simulink model "HeliControl_with_UDE_R2018a"  (Simulink 9.1)
settings: Solver=ode3  StartTime=0.0  StopTime=50  FixedStep=0.005  RelTol=1e-3
StopFcn:
  | %save('data.mat','ans_eps','ans_eps_d','ans_psi','ans_psi_d','ans_theta','ans_theta_d','u_ele','u_psi','u_theta','dhat_ele','dhat_psi','dhat_theta')
values from neighbouring files (symbols this model uses):
  a1 = 0.2634    [init_simulation.m]
  a2 = 1.6279    [init_simulation.m]
  a3 = 25.6488    [init_simulation.m]
  b1 = 0.531    [init_simulation.m]
  b2 = 5.3292    [init_simulation.m]
  b3 = 0.531    [init_simulation.m]
  b4 = 0.1157    [init_simulation.m]
  ce = 0.3010    (= 0.301)    [init_simulation.m]
  cp = 0.6804    [init_simulation.m]
  ct = 0.3410    (= 0.341)    [init_simulation.m]
  k_double_epsilon = [ ki_epsilon  kp_epsilon   kd_epsilon ]    [init_simulation.m]
  k_double_psi = [ki_psi   kp_psi    kd_psi]    [init_simulation.m]
  k_double_theta = [ki_theta   kp_theta   kd_theta]    [init_simulation.m]
  n = 0.9    [init_simulation.m]
  w = 125.66    [init_simulation.m]
undefined symbols (not defined in the file or in its folder): epsilon_T, psi_T, theta_T
libraries: powerlib_extras x1
settings Model: Creator=5420  LastModifiedBy=LaVie  ExtModeTrigDuration=200000
settings DataIOCC: LimitDataPoints=on  SignalLoggingSaveFormat=ModelDataLogs  SignalLoggingName=sigsOut
settings OptimizationCC: ExpressionDepthLimit=2147483647  InitFltsAndDblsToZero=on  LifeSpan=auto
settings DebuggingCC: SaveWithParameterizedLinksMsg=none  SignalResolutionControl=TryResolveAllWithWarning  MultiTaskDSMMsg=warning  MultiTaskCondExecSysMsg=none  StateNameClashWarn=warning
settings HardwareCC: ProdBitPerLong=64  ProdBitPerPointer=64  ProdBitPerSizeT=64  ProdBitPerPtrDiffT=64  ProdLargestAtomicFloat=Float  ProdIntDivRoundTo=Zero  ProdEndianess=LittleEndian  ProdWordSize=64  ProdHWDeviceType=Intel->x86-64 (Linux 64)
settings RTWCC: Description=Simulink Desktop Real-Time  SystemTargetFile=sldrt.tlc  TemplateMakefile=sldrt.tmf  RTWCompilerOptimization=on
settings CodeAppCC: MaxIdLength=95
settings SimulinkDesktopRealTimeCC: TargetLibSuffix=_sldrt.a  TargetPreCompLibLocation=E:\matlab2022a\toolbox\sldrt\lib\win64  TargetLangStandard=C89/C90 (ANSI)  ModelReferenceCompliant=off  CompOptLevelCompliant=off  SupportVariableSizeSignals=off

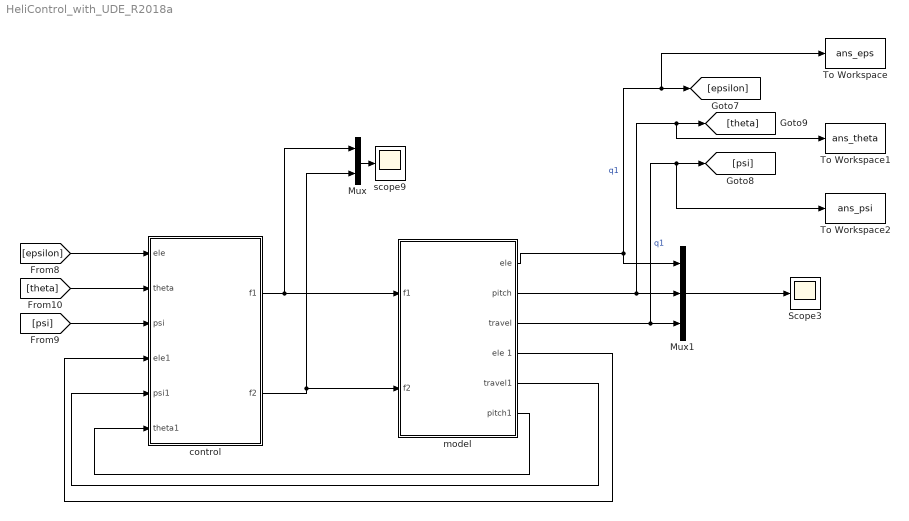
== system HeliControl_with_UDE_R2018a ==
  Mux : Mux  Inputs=2
  Mux1 : Mux  Inputs=3
  Scope3 : Scope
  To Workspace : ToWorkspace  VariableName=ans_eps  SaveFormat=Structure With Time  SampleTime=-1
      settings: Save2DSignal=2-D array (concatenate along first dimension)
  To Workspace1 : ToWorkspace  VariableName=ans_theta  SampleTime=-1
      settings: Save2DSignal=2-D array (concatenate along first dimension)
  To Workspace2 : ToWorkspace  VariableName=ans_psi  SampleTime=-1
      settings: Save2DSignal=2-D array (concatenate along first dimension)
  control : Subsystem
  model : Subsystem
  scope9 : Scope
  wires:
  Mux1/1 -> Scope3/1
  control/2(f2) -> Mux/2, model/2(f2)
  control/1(f1) -> Mux/1, model/1(f1)
  [epsilon] -> control/1(ele)
  [theta] -> control/2(theta)
  [psi] -> control/3(psi)
  Mux/1 -> scope9/1
  model/1("ele ") -> To Workspace/1, [epsilon], Mux1/1  "q1"
  model/2(pitch) -> To Workspace1/1, [theta], Mux1/2
  model/3(travel) -> To Workspace2/1, [psi], Mux1/3  "q1"
  model/4(ele 1) -> control/4(ele1)
  model/5(travel1) -> control/5(psi1)
  model/6(pitch1) -> control/6(theta1)

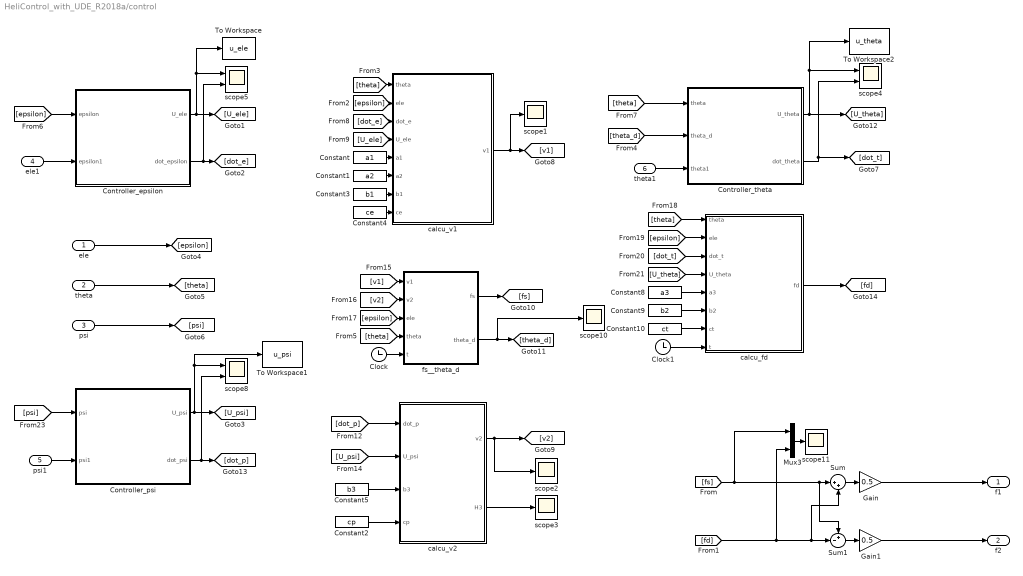
== system HeliControl_with_UDE_R2018a/control ==
  ele : Inport
  theta : Inport  Port=2
  psi : Inport  Port=3
  ele1 : Inport  Port=4
  psi1 : Inport  Port=5
  theta1 : Inport  Port=6
  Clock : Clock
      settings: Decimation=30
  Clock1 : Clock
      settings: Decimation=30
  Constant : Constant  Value=a1
  Constant1 : Constant  Value=a2
  Constant10 : Constant  Value=ct
  Constant2 : Constant  Value=cp
  Constant3 : Constant  Value=b1
  Constant4 : Constant  Value=ce
  Constant5 : Constant  Value=b3
  Constant8 : Constant  Value=a3
  Constant9 : Constant  Value=b2
  Controller_epsilon : Subsystem
  Controller_psi : Subsystem
  Controller_theta : Subsystem
  Gain : Gain  Gain=0.5
  Gain1 : Gain  Gain=0.5
  Mux3 : Mux  Inputs=2
  Sum : Sum  Inputs=|++
  Sum1 : Sum  Inputs=+-|
  To Workspace : ToWorkspace  VariableName=u_ele  SampleTime=-1
      settings: Save2DSignal=2-D array (concatenate along first dimension)
  To Workspace1 : ToWorkspace  VariableName=u_psi  SampleTime=-1
      settings: Save2DSignal=2-D array (concatenate along first dimension)
  To Workspace2 : ToWorkspace  VariableName=u_theta  SampleTime=-1
      settings: Save2DSignal=2-D array (concatenate along first dimension)
  calcu_fd : MATLAB Function  TreatAsAtomicUnit=on
  calcu_v1 : MATLAB Function  TreatAsAtomicUnit=on
  calcu_v2 : MATLAB Function  TreatAsAtomicUnit=on
  fs__theta_d : MATLAB Function  TreatAsAtomicUnit=on
  scope{1..3,10..11} (5 alike) : Scope
  scope4 : Scope  NumInputPorts=2
  scope5 : Scope  NumInputPorts=2
  scope8 : Scope  NumInputPorts=2
  f1 : Outport  VectorParamsAs1DForOutWhenUnconnected=off
  f2 : Outport  Port=2  VectorParamsAs1DForOutWhenUnconnected=off
  wires:
  [theta] -> calcu_v1/1(theta)
  [epsilon] -> calcu_v1/2(ele)
  calcu_v2/1(v2) -> [v2], scope2/1
  [U_ele] -> calcu_v1/4(U_ele)
  [dot_e] -> calcu_v1/3(dot_e)
  calcu_v1/1(v1) -> scope1/1, [v1]
  [v1] -> fs__theta_d/1(v1)
  [v2] -> fs__theta_d/2(v2)
  [epsilon] -> fs__theta_d/3(ele)
  fs__theta_d/1(fs) -> [fs]
  fs__theta_d/2(theta_d) -> scope10/1, [theta_d]
  [theta] -> calcu_fd/1(theta)
  [epsilon] -> calcu_fd/2(ele)
  [dot_t] -> calcu_fd/3(dot_t)
  [U_theta] -> calcu_fd/4(U_theta)
  calcu_fd/1(fd) -> [fd]
  [fd] -> Sum/2, Sum1/2, Mux3/2
  Sum/1 -> Gain/1
  Sum1/1 -> Gain1/1
  ele/1 -> [epsilon]
  theta/1 -> [theta]
  psi/1 -> [psi]
  Mux3/1 -> scope11/1
  Constant/1 -> calcu_v1/5(a1)
  Constant1/1 -> calcu_v1/6(a2)
  Constant3/1 -> calcu_v1/7(b1)
  Constant4/1 -> calcu_v1/8(ce)
  Constant8/1 -> calcu_fd/5(a3)
  Constant9/1 -> calcu_fd/6(b2)
  Constant10/1 -> calcu_fd/7(ct)
  [theta] -> fs__theta_d/4(theta)
  Clock/1 -> fs__theta_d/5(t)
  Clock1/1 -> calcu_fd/8(t)
  calcu_v2/2(H3) -> scope3/1
  [epsilon] -> Controller_epsilon/1(epsilon)
  Controller_epsilon/2(dot_epsilon) -> scope5/2, [dot_e]
  [psi] -> Controller_psi/1(psi)
  Controller_psi/1(U_psi) -> scope8/1, To Workspace1/1, [U_psi]
  Controller_psi/2(dot_psi) -> scope8/2, [dot_p]
  [theta] -> Controller_theta/1(theta)
  Controller_theta/1(U_theta) -> To Workspace2/1, scope4/1, [U_theta]
  Controller_theta/2(dot_theta) -> scope4/2, [dot_t]
  [theta_d] -> Controller_theta/2(theta_d)
  Controller_epsilon/1(U_ele) -> To Workspace/1, scope5/1, [U_ele]
  ele1/1 -> Controller_epsilon/2(epsilon1)
  psi1/1 -> Controller_psi/2(psi1)
  theta1/1 -> Controller_theta/3(theta1)
  Gain/1 -> f1/1
  Gain1/1 -> f2/1
  [fs] -> Sum1/1, Sum/1, Mux3/1
  [dot_p] -> calcu_v2/1(dot_p)
  [U_psi] -> calcu_v2/2(U_psi)
  Constant5/1 -> calcu_v2/3(b3)
  Constant2/1 -> calcu_v2/4(cp)

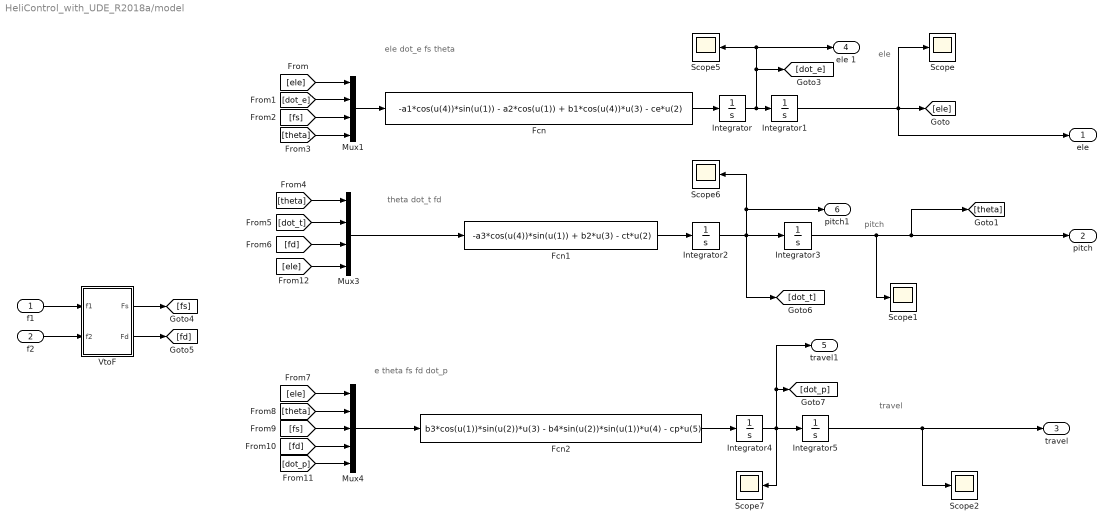
== system HeliControl_with_UDE_R2018a/model ==
  note: e
      | theta
      | fs
      | fd
      | dot_p
  note: ele
      | dot_e
      | fs
      | theta
  note: travel
  note: pitch
  note: ele
  note: theta
      | dot_t
      | fd
  f1 : Inport
  f2 : Inport  Port=2
  Fcn : Fcn  Expr=-a1*cos(u(4))*sin(u(1)) - a2*cos(u(1)) + b1*cos(u(4))*u(3) - ce*u(2)
  Fcn1 : Fcn  Expr=-a3*cos(u(4))*sin(u(1)) + b2*u(3) - ct*u(2)
  Fcn2 : Fcn  Expr=b3*cos(u(1))*sin(u(2))*u(3) - b4*sin(u(2))*sin(u(1))*u(4) - cp*u(5)
  Integrator{,2..5} (5 alike) : Integrator
  Integrator1 : Integrator  InitialCondition=-0.713
  Mux1 : Mux
  Mux3 : Mux
  Mux4 : Mux  Inputs=5
  Scope{,1..2,5..7} (6 alike) : Scope
  VtoF : Subsystem
  "ele " : Outport  VectorParamsAs1DForOutWhenUnconnected=off
  pitch : Outport  Port=2  VectorParamsAs1DForOutWhenUnconnected=off
  travel : Outport  Port=3  VectorParamsAs1DForOutWhenUnconnected=off
  ele 1 : Outport  Port=4  VectorParamsAs1DForOutWhenUnconnected=off
  travel1 : Outport  Port=5  VectorParamsAs1DForOutWhenUnconnected=off
  pitch1 : Outport  Port=6  VectorParamsAs1DForOutWhenUnconnected=off
  wires:
  Integrator1/1 -> "ele "/1, Scope/1, [ele]
  Fcn/1 -> Integrator/1
  Integrator3/1 -> pitch/1, [theta], Scope1/1
  Integrator/1 -> ele 1/1, Scope5/1, [dot_e], Integrator1/1
  Fcn1/1 -> Integrator2/1
  Fcn2/1 -> Integrator4/1
  Integrator4/1 -> Scope7/1, travel1/1, [dot_p], Integrator5/1
  Integrator5/1 -> travel/1, Scope2/1
  Mux1/1 -> Fcn/1
  Mux4/1 -> Fcn2/1
  [ele] -> Mux1/1
  [dot_e] -> Mux1/2
  VtoF/1(Fs) -> [fs]
  VtoF/2(Fd) -> [fd]
  [fs] -> Mux1/3
  [theta] -> Mux1/4
  [ele] -> Mux4/1
  [theta] -> Mux4/2
  [fs] -> Mux4/3
  [fd] -> Mux4/4
  [dot_p] -> Mux4/5
  Integrator2/1 -> Scope6/1, pitch1/1, [dot_t], Integrator3/1
  f1/1 -> VtoF/1(f1)
  f2/1 -> VtoF/2(f2)
  Mux3/1 -> Fcn1/1
  [theta] -> Mux3/1
  [dot_t] -> Mux3/2
  [fd] -> Mux3/3
  [ele] -> Mux3/4

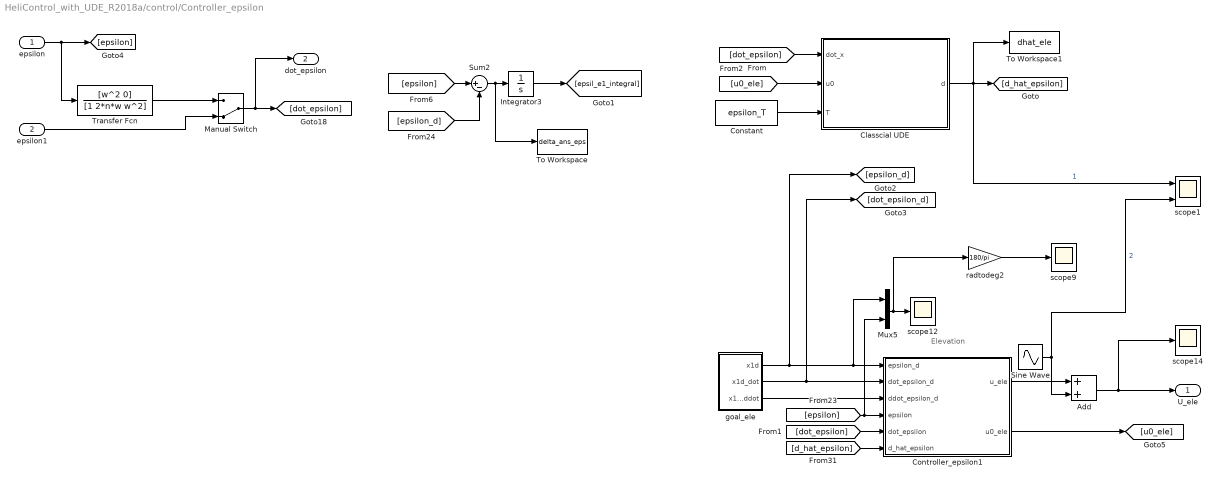
== system HeliControl_with_UDE_R2018a/control/Controller_epsilon ==
  note: Elevation
  epsilon : Inport
  epsilon1 : Inport  Port=2
  Add : Sum
  Classcial UDE : Subsystem
  Constant : Constant  Value=epsilon_T  VectorParams1D=off  SampleTime=-1
  Controller_epsilon1 : Subsystem
  Integrator3 : Integrator
  Manual Switch : ManualSwitch  CurrentSetting=0
  Mux5 : Mux  Inputs=2
  Sine Wave : Sin  Amplitude=0.05  Bias=0.1  Frequency=0.5  SampleTime=0
  Sum2 : Sum  Inputs=|+-
  To Workspace : ToWorkspace  VariableName=delta_ans_eps  SaveFormat=Timeseries  SampleTime=-1
  To Workspace1 : ToWorkspace  VariableName=dhat_ele  SampleTime=-1
      settings: Save2DSignal=2-D array (concatenate along first dimension)
  Transfer Fcn : TransferFcn  Numerator=[w^2 0]  Denominator=[1 2*n*w w^2]
  goal_ele : Subsystem
  radtodeg2 : Gain  Gain=180/pi
  scope1 : Scope  NumInputPorts=2
  scope12 : Scope
  scope14 : Scope
  scope9 : Scope
  U_ele : Outport  VectorParamsAs1DForOutWhenUnconnected=off
  dot_epsilon : Outport  Port=2  VectorParamsAs1DForOutWhenUnconnected=off
  wires:
  [epsilon] -> Controller_epsilon1/4(epsilon), Mux5/2
  Mux5/1 -> radtodeg2/1, scope12/1
  Add/1 -> scope14/1, U_ele/1
  radtodeg2/1 -> scope9/1
  goal_ele/1(x1d) -> Mux5/1, Controller_epsilon1/1(epsilon_d), [epsilon_d]
  goal_ele/2(x1d_dot) -> [dot_epsilon_d], Controller_epsilon1/2(dot_epsilon_d)
  goal_ele/3(x1d_ddot) -> Controller_epsilon1/3(ddot_epsilon_d)
  Sum2/1 -> To Workspace/1, Integrator3/1
  Integrator3/1 -> [epsil_e1_integral]
  [epsilon_d] -> Sum2/2
  [epsilon] -> Sum2/1
  [d_hat_epsilon] -> Controller_epsilon1/6(d_hat_epsilon)
  epsilon/1 -> Transfer Fcn/1, [epsilon]
  [dot_epsilon] -> Controller_epsilon1/5(dot_epsilon)
  Transfer Fcn/1 -> Manual Switch/1
  Manual Switch/1 -> dot_epsilon/1, [dot_epsilon]
  epsilon1/1 -> Manual Switch/2
  Controller_epsilon1/2(u0_ele) -> [u0_ele]
  Classcial UDE/1(d) -> scope1/1, To Workspace1/1, [d_hat_epsilon]  "1"
  [dot_epsilon] -> Classcial UDE/1(dot_x)
  [u0_ele] -> Classcial UDE/2(u0)
  Constant/1 -> Classcial UDE/3(T)
  Controller_epsilon1/1(u_ele) -> Add/1
  Sine Wave/1 -> Add/2, scope1/2  "2"

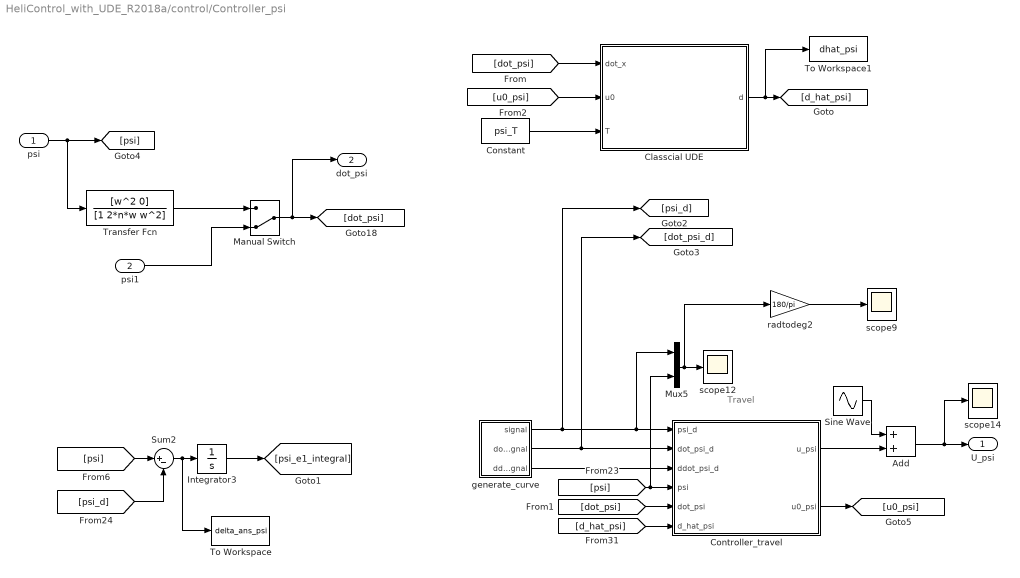
== system HeliControl_with_UDE_R2018a/control/Controller_psi ==
  note: Travel
  psi : Inport
  psi1 : Inport  Port=2
  Add : Sum
  Classcial UDE : Subsystem
  Constant : Constant  Value=psi_T  VectorParams1D=off  SampleTime=-1
  Controller_travel : Subsystem
  Integrator3 : Integrator
  Manual Switch : ManualSwitch  CurrentSetting=0
  Mux5 : Mux  Inputs=2
  Sine Wave : Sin  Amplitude=0.05  Bias=0.1  Frequency=2  SampleTime=0
  Sum2 : Sum  Inputs=|+-
  To Workspace : ToWorkspace  VariableName=delta_ans_psi  SaveFormat=Timeseries  SampleTime=-1
  To Workspace1 : ToWorkspace  VariableName=dhat_psi  SampleTime=-1
      settings: Save2DSignal=2-D array (concatenate along first dimension)
  Transfer Fcn : TransferFcn  Numerator=[w^2 0]  Denominator=[1 2*n*w w^2]
  generate_curve : Subsystem
  radtodeg2 : Gain  Gain=180/pi
  scope12 : Scope
  scope14 : Scope
  scope9 : Scope
  U_psi : Outport  VectorParamsAs1DForOutWhenUnconnected=off
  dot_psi : Outport  Port=2  VectorParamsAs1DForOutWhenUnconnected=off
  wires:
  [psi] -> Controller_travel/4(psi), Mux5/2
  Mux5/1 -> radtodeg2/1, scope12/1
  Add/1 -> U_psi/1, scope14/1
  radtodeg2/1 -> scope9/1
  generate_curve/1(signal) -> Mux5/1, Controller_travel/1(psi_d), [psi_d]
  generate_curve/2(dot_signal) -> [dot_psi_d], Controller_travel/2(dot_psi_d)
  generate_curve/3(ddot_signal) -> Controller_travel/3(ddot_psi_d)
  Sum2/1 -> To Workspace/1, Integrator3/1
  Integrator3/1 -> [psi_e1_integral]
  [psi_d] -> Sum2/2
  [psi] -> Sum2/1
  [d_hat_psi] -> Controller_travel/6(d_hat_psi)
  psi/1 -> Transfer Fcn/1, [psi]
  [dot_psi] -> Controller_travel/5(dot_psi)
  Transfer Fcn/1 -> Manual Switch/1
  Manual Switch/1 -> dot_psi/1, [dot_psi]
  psi1/1 -> Manual Switch/2
  [dot_psi] -> Classcial UDE/1(dot_x)
  Classcial UDE/1(d) -> To Workspace1/1, [d_hat_psi]
  [u0_psi] -> Classcial UDE/2(u0)
  Constant/1 -> Classcial UDE/3(T)
  Controller_travel/2(u0_psi) -> [u0_psi]
  Sine Wave/1 -> Add/1
  Controller_travel/1(u_psi) -> Add/2

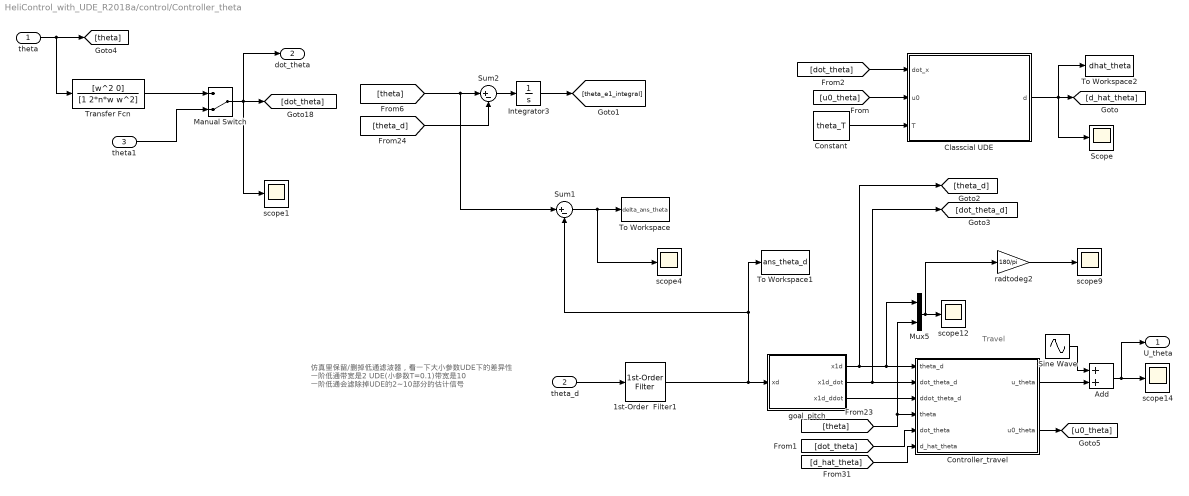
== system HeliControl_with_UDE_R2018a/control/Controller_theta ==
  note: 仿真里保留/删掉低通滤波器，看一下大小参数UDE下的差异性
      | 一阶低通带宽是2
      | UDE(小参数T=0.1)带宽是10
      | 一阶低通会滤除掉UDE的2~10部分的估计信号
  note: Travel
  theta : Inport
  theta_d : Inport  Port=2
  theta1 : Inport  Port=3
  1st-Order  Filter1 : powerlib_extras/Control  Blocks/1st-Order  Filter  FilterType=Lowpass  Tc=0.5  Initialize=off  Vac_Init=[0.8 -25 60]  Vdc_Init=-0.4  PlotResponse=off  param1=[1 500 1]
      settings: SourceProductBaseCode=PS
  Add : Sum
  Classcial UDE : Subsystem
  Constant : Constant  Value=theta_T  VectorParams1D=off  SampleTime=-1
  Controller_travel : Subsystem
  Integrator3 : Integrator
  Manual Switch : ManualSwitch  CurrentSetting=0
  Mux5 : Mux  Inputs=2
  Scope : Scope
  Sine Wave : Sin  Amplitude=0.05  Bias=0.1  Frequency=5  SampleTime=0
  Sum1 : Sum  Inputs=|+-
  Sum2 : Sum  Inputs=|+-
  To Workspace : ToWorkspace  VariableName=delta_ans_theta  SaveFormat=Timeseries  SampleTime=-1
  To Workspace1 : ToWorkspace  VariableName=ans_theta_d  SampleTime=-1
      settings: Save2DSignal=2-D array (concatenate along first dimension)
  To Workspace2 : ToWorkspace  VariableName=dhat_theta  SampleTime=-1
      settings: Save2DSignal=2-D array (concatenate along first dimension)
  Transfer Fcn : TransferFcn  Numerator=[w^2 0]  Denominator=[1 2*n*w w^2]
  goal_pitch : Subsystem
  radtodeg2 : Gain  Gain=180/pi
  scope{1,4,9,12,14} (5 alike) : Scope
  U_theta : Outport  VectorParamsAs1DForOutWhenUnconnected=off
  dot_theta : Outport  Port=2  VectorParamsAs1DForOutWhenUnconnected=off
  wires:
  [theta] -> Controller_travel/4(theta), Mux5/2
  Mux5/1 -> radtodeg2/1, scope12/1
  Add/1 -> scope14/1, U_theta/1
  radtodeg2/1 -> scope9/1
  goal_pitch/1(x1d) -> Mux5/1, Controller_travel/1(theta_d), [theta_d]
  goal_pitch/2(x1d_dot) -> [dot_theta_d], Controller_travel/2(dot_theta_d)
  goal_pitch/3(x1d_ddot) -> Controller_travel/3(ddot_theta_d)
  Sum2/1 -> Integrator3/1
  Integrator3/1 -> [theta_e1_integral]
  [theta_d] -> Sum2/2
  [d_hat_theta] -> Controller_travel/6(d_hat_theta)
  theta/1 -> Transfer Fcn/1, [theta]
  [dot_theta] -> Controller_travel/5(dot_theta)
  Transfer Fcn/1 -> Manual Switch/1
  Manual Switch/1 -> scope1/1, dot_theta/1, [dot_theta]
  theta1/1 -> Manual Switch/2
  [theta] -> Sum1/1, Sum2/1
  Sum1/1 -> scope4/1, To Workspace/1
  1st-Order  Filter1/1 -> goal_pitch/1(xd), To Workspace1/1, Sum1/2
  Controller_travel/2(u0_theta) -> [u0_theta]
  [u0_theta] -> Classcial UDE/2(u0)
  Classcial UDE/1(d) -> Scope/1, To Workspace2/1, [d_hat_theta]
  [dot_theta] -> Classcial UDE/1(dot_x)
  Constant/1 -> Classcial UDE/3(T)
  Sine Wave/1 -> Add/1
  Controller_travel/1(u_theta) -> Add/2
  theta_d/1 -> 1st-Order  Filter1/1

== system HeliControl_with_UDE_R2018a/model/VtoF ==
  f1 : Inport
  f2 : Inport  Port=2
  Add : Sum
  Add1 : Sum  Inputs=+-
  Fs : Outport  VectorParamsAs1DForOutWhenUnconnected=off
  Fd : Outport  Port=2  VectorParamsAs1DForOutWhenUnconnected=off
  wires:
  Add1/1 -> Fd/1
  f2/1 -> Add1/2, Add/2
  f1/1 -> Add1/1, Add/1
  Add/1 -> Fs/1

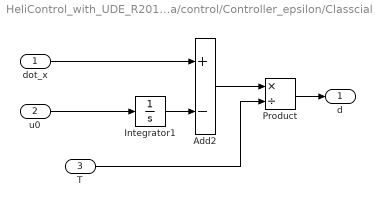
== system HeliControl_with_UDE_R2018a/control/Controller_epsilon/Classcial UDE ==
  dot_x : Inport
  u0 : Inport  Port=2
  T : Inport  Port=3
  Add2 : Sum  Inputs=+-
  Integrator1 : Integrator
  Product : Product  Inputs=*/
  d : Outport  VectorParamsAs1DForOutWhenUnconnected=off
  wires:
  dot_x/1 -> Add2/1
  Integrator1/1 -> Add2/2
  u0/1 -> Integrator1/1
  Add2/1 -> Product/1
  Product/1 -> d/1
  T/1 -> Product/2

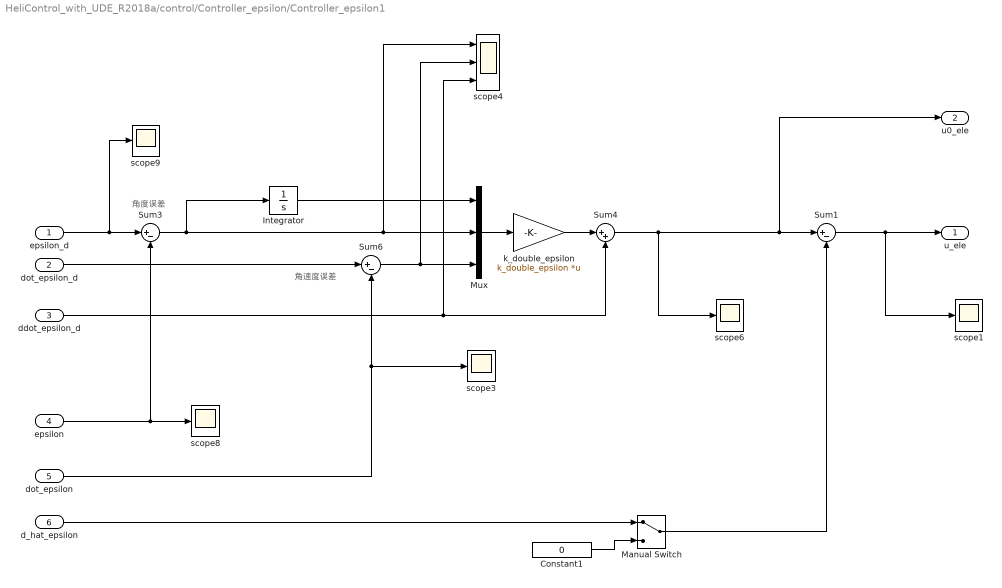
== system HeliControl_with_UDE_R2018a/control/Controller_epsilon/Controller_epsilon1 ==
  note: 角速度误差
  note: 角度误差
  epsilon_d : Inport
  dot_epsilon_d : Inport  Port=2
  ddot_epsilon_d : Inport  Port=3
  epsilon : Inport  Port=4
  dot_epsilon : Inport  Port=5
  d_hat_epsilon : Inport  Port=6
  Constant1 : Constant  Value=0
  Integrator : Integrator
  Manual Switch : ManualSwitch
  Mux : Mux  Inputs=3
  Sum1 : Sum  Inputs=|+-
  Sum3 : Sum  Inputs=|+-
  Sum4 : Sum  Inputs=|++
  Sum6 : Sum  Inputs=|+-
  k_double_epsilon : Gain  Gain=k_double_epsilon  Multiplication=Matrix(K*u)
  scope{1,3,6,8..9} (5 alike) : Scope
  scope4 : Scope  NumInputPorts=3
  u_ele : Outport  VectorParamsAs1DForOutWhenUnconnected=off
  u0_ele : Outport  Port=2  VectorParamsAs1DForOutWhenUnconnected=off
  wires:
  epsilon/1 -> Sum3/2, scope8/1
  epsilon_d/1 -> scope9/1, Sum3/1
  Sum4/1 -> u0_ele/1, Sum1/1, scope6/1
  Sum3/1 -> scope4/1, Mux/2, Integrator/1
  Sum6/1 -> scope4/2, Mux/3
  Mux/1 -> k_double_epsilon/1
  dot_epsilon_d/1 -> Sum6/1
  k_double_epsilon/1 -> Sum4/1
  ddot_epsilon_d/1 -> scope4/3, Sum4/2
  dot_epsilon/1 -> Sum6/2, scope3/1
  Integrator/1 -> Mux/1
  Sum1/1 -> scope1/1, u_ele/1
  Manual Switch/1 -> Sum1/2
  d_hat_epsilon/1 -> Manual Switch/1
  Constant1/1 -> Manual Switch/2

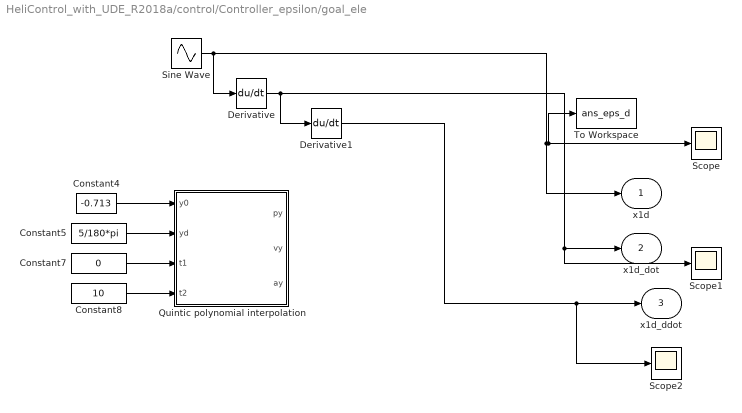
== system HeliControl_with_UDE_R2018a/control/Controller_epsilon/goal_ele ==
  Constant4 : Constant  Value=-0.713  VectorParams1D=off  SampleTime=-1
  Constant5 : Constant  Value=5/180*pi  VectorParams1D=off  SampleTime=-1
  Constant7 : Constant  Value=0  VectorParams1D=off  SampleTime=-1
  Constant8 : Constant  Value=10  VectorParams1D=off  SampleTime=-1
  Derivative : Derivative
  Derivative1 : Derivative
  Quintic polynomial interpolation : Subsystem
  Scope : Scope
  Scope1 : Scope
  Scope2 : Scope
  Sine Wave : Sin  Amplitude=-2*pi/180  Bias=2*pi/180  Frequency=0.4*pi  Phase=pi/2  SampleTime=0
  To Workspace : ToWorkspace  VariableName=ans_eps_d  SampleTime=-1
      settings: Save2DSignal=2-D array (concatenate along first dimension)
  x1d : Outport  VectorParamsAs1DForOutWhenUnconnected=off
  x1d_dot : Outport  Port=2  VectorParamsAs1DForOutWhenUnconnected=off
  x1d_ddot : Outport  Port=3  VectorParamsAs1DForOutWhenUnconnected=off
  wires:
  Derivative1/1 -> Scope2/1, x1d_ddot/1
  Derivative/1 -> Derivative1/1, Scope1/1, x1d_dot/1
  Sine Wave/1 -> Derivative/1, x1d/1, To Workspace/1, Scope/1
  Constant4/1 -> Quintic polynomial interpolation/1(y0)
  Constant5/1 -> Quintic polynomial interpolation/2(yd)
  Constant7/1 -> Quintic polynomial interpolation/3(t1)
  Constant8/1 -> Quintic polynomial interpolation/4(t2)

== system HeliControl_with_UDE_R2018a/control/Controller_psi/Classcial UDE ==
  dot_x : Inport
  u0 : Inport  Port=2
  T : Inport  Port=3
  Add2 : Sum  Inputs=+-
  Integrator1 : Integrator
  Product : Product  Inputs=*/
  d : Outport  VectorParamsAs1DForOutWhenUnconnected=off
  wires:
  dot_x/1 -> Add2/1
  Integrator1/1 -> Add2/2
  u0/1 -> Integrator1/1
  Add2/1 -> Product/1
  Product/1 -> d/1
  T/1 -> Product/2

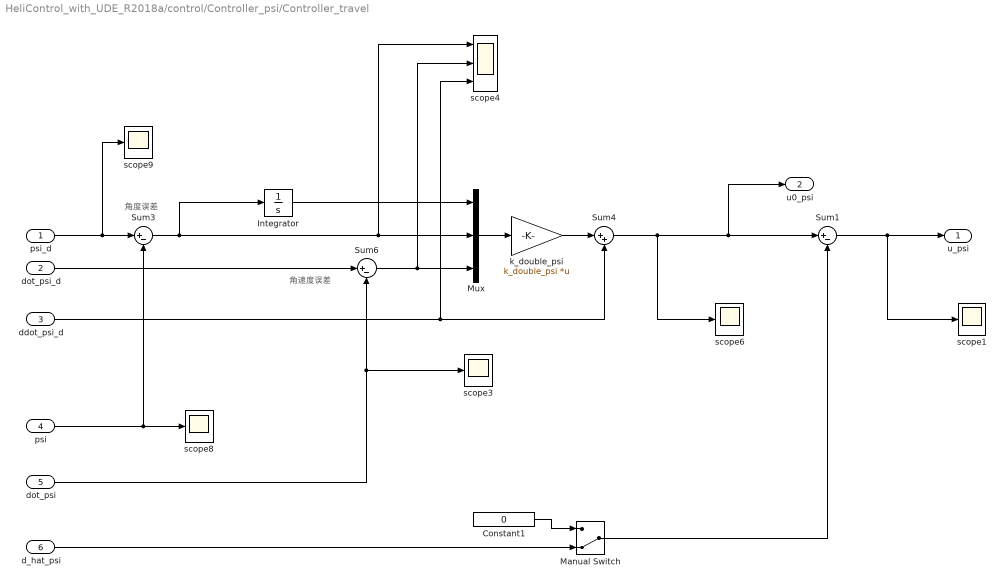
== system HeliControl_with_UDE_R2018a/control/Controller_psi/Controller_travel ==
  note: 角速度误差
  note: 角度误差
  psi_d : Inport
  dot_psi_d : Inport  Port=2
  ddot_psi_d : Inport  Port=3
  psi : Inport  Port=4
  dot_psi : Inport  Port=5
  d_hat_psi : Inport  Port=6
  Constant1 : Constant  Value=0
  Integrator : Integrator
  Manual Switch : ManualSwitch  CurrentSetting=0
  Mux : Mux  Inputs=3
  Sum1 : Sum  Inputs=|+-
  Sum3 : Sum  Inputs=|+-
  Sum4 : Sum  Inputs=|++
  Sum6 : Sum  Inputs=|+-
  k_double_psi : Gain  Gain=k_double_psi  Multiplication=Matrix(K*u)
  scope{1,3,6,8..9} (5 alike) : Scope
  scope4 : Scope  NumInputPorts=3
  u_psi : Outport  VectorParamsAs1DForOutWhenUnconnected=off
  u0_psi : Outport  Port=2  VectorParamsAs1DForOutWhenUnconnected=off
  wires:
  psi/1 -> Sum3/2, scope8/1
  psi_d/1 -> scope9/1, Sum3/1
  Sum4/1 -> u0_psi/1, Sum1/1, scope6/1
  Sum3/1 -> scope4/1, Mux/2, Integrator/1
  Sum6/1 -> scope4/2, Mux/3
  Mux/1 -> k_double_psi/1
  dot_psi_d/1 -> Sum6/1
  k_double_psi/1 -> Sum4/1
  ddot_psi_d/1 -> scope4/3, Sum4/2
  dot_psi/1 -> Sum6/2, scope3/1
  Integrator/1 -> Mux/1
  Sum1/1 -> scope1/1, u_psi/1
  Constant1/1 -> Manual Switch/1
  d_hat_psi/1 -> Manual Switch/2
  Manual Switch/1 -> Sum1/2

== system HeliControl_with_UDE_R2018a/control/Controller_psi/generate_curve ==
  Clock : Clock
  Constant1 : Constant  Value=0  VectorParams1D=off  SampleTime=-1
  MATLAB Function : MATLAB Function  TreatAsAtomicUnit=on
  To Workspace : ToWorkspace  VariableName=ans_psi_d  SampleTime=-1
      settings: Save2DSignal=2-D array (concatenate along first dimension)
  signal : Outport  VectorParamsAs1DForOutWhenUnconnected=off
  dot_signal : Outport  Port=2  VectorParamsAs1DForOutWhenUnconnected=off
  ddot_signal : Outport  Port=3  VectorParamsAs1DForOutWhenUnconnected=off
  wires:
  MATLAB Function/1(p) -> To Workspace/1, signal/1
  MATLAB Function/2(v) -> dot_signal/1
  Constant1/1 -> ddot_signal/1
  Clock/1 -> MATLAB Function/1(t)

== system HeliControl_with_UDE_R2018a/control/Controller_theta/Classcial UDE ==
  dot_x : Inport
  u0 : Inport  Port=2
  T : Inport  Port=3
  Add2 : Sum  Inputs=+-
  Integrator1 : Integrator
  Product : Product  Inputs=*/
  d : Outport  VectorParamsAs1DForOutWhenUnconnected=off
  wires:
  dot_x/1 -> Add2/1
  Integrator1/1 -> Add2/2
  u0/1 -> Integrator1/1
  Add2/1 -> Product/1
  Product/1 -> d/1
  T/1 -> Product/2

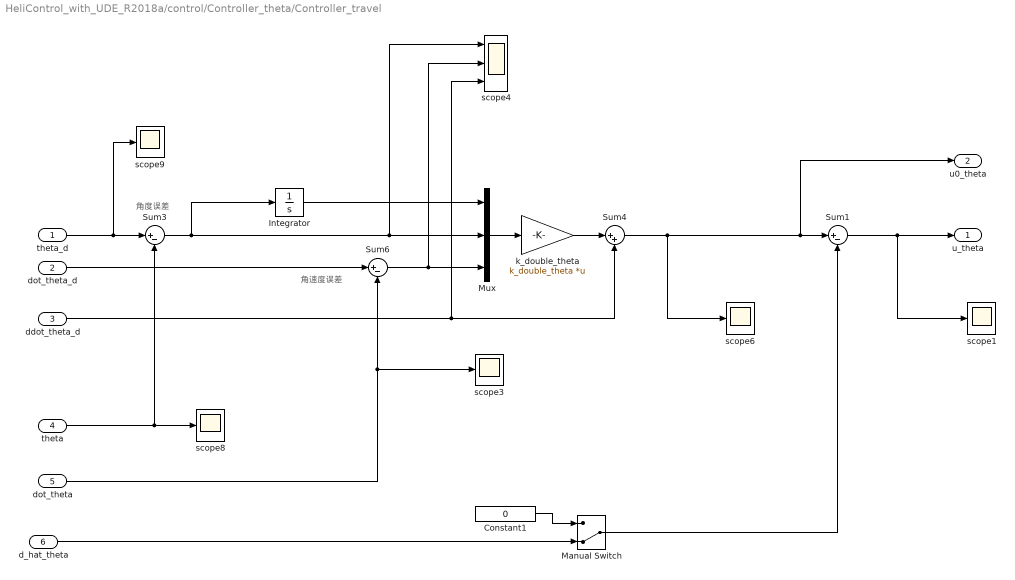
== system HeliControl_with_UDE_R2018a/control/Controller_theta/Controller_travel ==
  note: 角速度误差
  note: 角度误差
  theta_d : Inport
  dot_theta_d : Inport  Port=2
  ddot_theta_d : Inport  Port=3
  theta : Inport  Port=4
  dot_theta : Inport  Port=5
  d_hat_theta : Inport  Port=6
  Constant1 : Constant  Value=0
  Integrator : Integrator
  Manual Switch : ManualSwitch  CurrentSetting=0
  Mux : Mux  Inputs=3
  Sum1 : Sum  Inputs=|+-
  Sum3 : Sum  Inputs=|+-
  Sum4 : Sum  Inputs=|++
  Sum6 : Sum  Inputs=|+-
  k_double_theta : Gain  Gain=k_double_theta  Multiplication=Matrix(K*u)
  scope{1,3,6,8..9} (5 alike) : Scope
  scope4 : Scope  NumInputPorts=3
  u_theta : Outport  VectorParamsAs1DForOutWhenUnconnected=off
  u0_theta : Outport  Port=2
  wires:
  theta/1 -> Sum3/2, scope8/1
  theta_d/1 -> scope9/1, Sum3/1
  Sum4/1 -> u0_theta/1, Sum1/1, scope6/1
  Sum3/1 -> scope4/1, Mux/2, Integrator/1
  Sum6/1 -> scope4/2, Mux/3
  Mux/1 -> k_double_theta/1
  dot_theta_d/1 -> Sum6/1
  k_double_theta/1 -> Sum4/1
  ddot_theta_d/1 -> scope4/3, Sum4/2
  dot_theta/1 -> Sum6/2, scope3/1
  Integrator/1 -> Mux/1
  Sum1/1 -> scope1/1, u_theta/1
  Constant1/1 -> Manual Switch/1
  d_hat_theta/1 -> Manual Switch/2
  Manual Switch/1 -> Sum1/2

== system HeliControl_with_UDE_R2018a/control/Controller_theta/goal_pitch ==
  xd : Inport
  Transfer Fcn1 : TransferFcn  Numerator=[w^2 0]  Denominator=[1 2*n*w w^2]
  Transfer Fcn2 : TransferFcn  Numerator=[w^2 0]  Denominator=[1 2*n*w w^2]
  scope1 : Scope
  x1d : Outport  VectorParamsAs1DForOutWhenUnconnected=off
  x1d_dot : Outport  Port=2  VectorParamsAs1DForOutWhenUnconnected=off
  x1d_ddot : Outport  Port=3  VectorParamsAs1DForOutWhenUnconnected=off
  wires:
  xd/1 -> Transfer Fcn1/1, scope1/1, x1d/1
  Transfer Fcn1/1 -> Transfer Fcn2/1, x1d_dot/1
  Transfer Fcn2/1 -> x1d_ddot/1

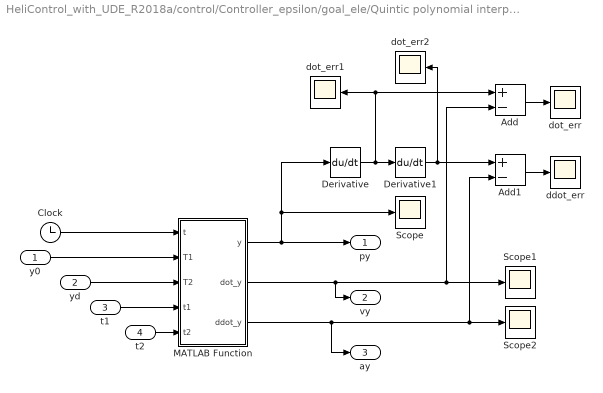
== system HeliControl_with_UDE_R2018a/control/Controller_epsilon/goal_ele/Quintic polynomial interpolation ==
  y0 : Inport
  yd : Inport  Port=2
  t1 : Inport  Port=3
  t2 : Inport  Port=4
  Add : Sum  Inputs=+-
  Add1 : Sum  Inputs=+-
  Clock : Clock
  Derivative : Derivative
  Derivative1 : Derivative
  MATLAB Function : MATLAB Function  TreatAsAtomicUnit=on
  Scope : Scope
  Scope1 : Scope
  Scope2 : Scope
  ddot_err : Scope
  dot_err : Scope
  dot_err1 : Scope
  dot_err2 : Scope
  py : Outport  VectorParamsAs1DForOutWhenUnconnected=off
  vy : Outport  Port=2  VectorParamsAs1DForOutWhenUnconnected=off
  ay : Outport  Port=3  VectorParamsAs1DForOutWhenUnconnected=off
  wires:
  Clock/1 -> MATLAB Function/1(t)
  MATLAB Function/1(y) -> py/1, Derivative/1, Scope/1
  y0/1 -> MATLAB Function/2(T1)
  yd/1 -> MATLAB Function/3(T2)
  t1/1 -> MATLAB Function/4(t1)
  t2/1 -> MATLAB Function/5(t2)
  MATLAB Function/2(dot_y) -> vy/1, Add/2, Scope1/1
  MATLAB Function/3(ddot_y) -> Add1/2, Scope2/1, ay/1
  Add/1 -> dot_err/1
  Derivative/1 -> Add/1, dot_err1/1, Derivative1/1
  Derivative1/1 -> dot_err2/1, Add1/1
  Add1/1 -> ddot_err/1

== matlab function control/calcu_v1 ==
  data: theta input double; v1 output double; ele input double; dot_e input double; U_ele input double; a1 input double; a2 input double; b1 input double; ce input double
function v1 = fcn(theta ,ele ,dot_e,U_ele   ,a1,a2,b1,ce)
%#codegen
H1 = -a1*cos(theta)*sin(ele)-a2*cos(ele)-ce*dot_e;
v1 = (U_ele-H1)/b1;

== matlab function control/Controller_psi/generate_curve/MATLAB Function ==
  data: t input double; p output double; v output double
function [p,v]= fcn(t)
    if t <= 10
        p = 0;
        v = 0;
    else
        if t<=35
            p = 2*pi/25*(t-10);
            v = 2*pi/25;
        else
            p = 2*pi;
            v = 0;
        end
    end
end

== matlab function control/calcu_v2 ==
  data: v2 output double; dot_p input double; U_psi input double; b3 input double; cp input double; H3 output double
function [v2,H3] = fcn(dot_p,U_psi,b3,cp)
%#fd is the diff_force of last time
% H3 = -b4*sin(theta)*sin(ele)*fd - cp*dot_p;
H3 = - cp*dot_p;
v2 = (U_psi-H3) /b3;

== matlab function control/fs__theta_d ==
  data: v1 input double; fs output double; v2 input double; ele input double; theta_d output double; theta input double; t input double
function [fs,theta_d] = fcn(v1,v2,ele,theta,t)
%7秒前仅有升降通道，俯仰及偏航不起作用
% if t>8
if t>0
fs = sqrt( v1^2 + (v2/cos(ele))^2 );
theta_d = atan( v2/(cos(ele)*v1) ); %rad

else
    fs = v1/cos(theta);
    theta_d = 0;
end

== matlab function control/calcu_fd ==
  data: theta input double; fd output double; ele input double; dot_t input double; U_theta input double; a3 input double; b2 input double; ct input double; t input double
function fd = fcn(theta ,ele ,dot_t,U_theta,a3,b2,ct,t)
%#codegen

% if t>8
if t>0
H2 = -a3*cos(ele)*sin(theta)-ct*dot_t;
fd = (U_theta-H2)/b2;

else
    fd = 0;
end

== matlab function control/Controller_epsilon/goal_ele/Quintic polynomial interpolation/MATLAB Function ==
  data: t input double; y output double; T1 input double; T2 input double; t1 input double; t2 input double; dot_y output double; ddot_y output double
function [y, dot_y, ddot_y] = fcn(t, T1, T2, t1, t2)
    a0 = T1;  % y(t1) 
    a1 = 0;  % dot_y(t1)
    a2 = 0;  % ddot_y(t1)/2
    a3 = 20*(T2-T1) / (2*(t2-t1)^3); 
    a4 = 30*(T1-T2) / (2*(t2-t1)^4);  
    a5 = 12*(T2-T1) / (2*(t2-t1)^5);

    u = t - t1;
    if u <= 0
        y = T1;
        dot_y = 0;
        ddot_y = 0;
    elseif u>0&&u<=(t2-t1)
        y = a0 + a1*u + a2*u^2 + a3*u^3 + a4*u^4 + a5*u^5;
        dot_y = a1 + 2*a2*u + 3*a3*u^2 + 4*a4*u^3 + 5*a5*u^4;
        ddot_y = 2*a2 + 6*a3*u + 12*a4*u^2 + 20*a5*u^3;
    else
        y = T2;
        dot_y = 0;
        ddot_y = 0;
    end

end
